simulink model "ten2"  (R2020b)
settings: Solver=VariableStepAuto  StartTime=0.0  StopTime=100  RelTol=1e-3
settings Model: Creator=20775  LastModifiedBy=20775

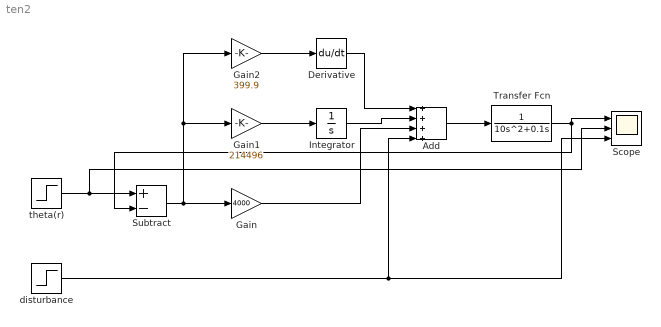
== system ten2 ==
  Add : Sum  Inputs=++++
  Derivative : Derivative
  Gain : Gain  Gain=4000
  Gain1 : Gain  Gain=214496
  Gain2 : Gain  Gain=399.9
  Integrator : Integrator
  Scope : Scope  NumInputPorts=3
  Subtract : Sum  Inputs=+-
  Transfer Fcn : TransferFcn  Denominator=[10 0.1 0]
  disturbance : Step  Time=40  After=20  SampleTime=0
  theta(r) : Step  Time=20  SampleTime=0
  wires:
  Transfer Fcn/1 -> Scope/1, Subtract/2
  Derivative/1 -> Add/1
  Integrator/1 -> Add/2
  Add/1 -> Transfer Fcn/1
  Gain2/1 -> Derivative/1
  Gain/1 -> Add/3
  Subtract/1 -> Gain2/1, Gain1/1, Gain/1
  theta(r)/1 -> Scope/2, Subtract/1
  Gain1/1 -> Integrator/1
  disturbance/1 -> Scope/3, Add/4
